simulink model "baseline_alt_vel_control"  (R2013a)
settings: Solver=FixedStepDiscrete  StartTime=0.0  StopTime=5  FixedStep=SampleTime  RelTol=1e-3
values from neighbouring files (symbols this model uses):
  ki_AT = 0.0017    [heading_gains.m]
  ki_VT = 0.02    [heading_gains.m]
  kp_AT = 0.021    [heading_gains.m]
  kp_VT = 0.091    [heading_gains.m]
  LP_filter = [0 0.0392;1 -.9608]    [heading_gains.m]
undefined symbols (not defined in the file or in its folder): AC, DiscIntNeverNeededParam, OperatingPoint, SampleTime, theta_sat, TrimCondition
libraries: Actuator_Lib x2, simulink x1, Controller_Lib x1
settings Model: Creator=austinmurch  LastModifiedBy=descobar
settings DataIOCC: SignalLoggingSaveFormat=ModelDataLogs
settings OptimizationCC: InlineParams=on  ExpressionDepthLimit=2147483647  SimCompilerOptimization=On
settings DebuggingCC: FcnCallInpInsideContextMsg=UseLocalSettings  StrictBusMsg=Warning
settings HardwareCC: ProdLargestAtomicInteger=Long  ProdLargestAtomicFloat=Double  ProdIntDivRoundTo=Zero  ProdEndianess=BigEndian  ProdHWDeviceType=Freescale->32-bit PowerPC
settings GRTTargetCC: CombineOutputUpdateFcns=off  GRTInterface=on

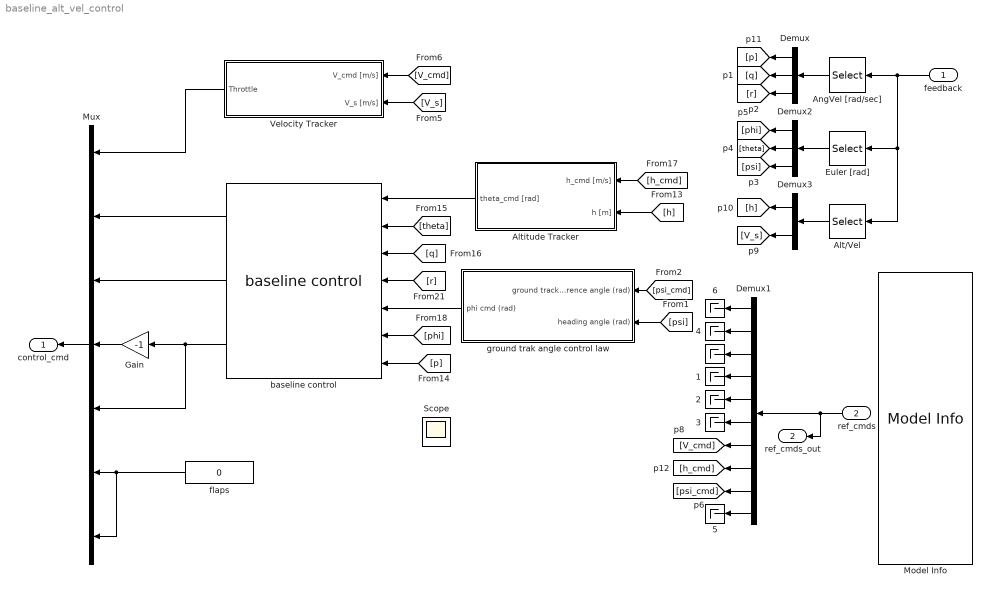
== system baseline_alt_vel_control ==
  feedback : Inport
  ref_cmds : Inport  Port=2
   {,1..6} (7 alike) : Terminator
  Alt/Vel : Selector  InputPortWidth=19  IndexOptions=Index vector (dialog)  Indices=[10:11]  OutputSizes=1
  Altitude Tracker : Subsystem
  AngVel [rad/sec] : Selector  InputPortWidth=19  IndexOptions=Index vector (dialog)  Indices=[4:6]  OutputSizes=1
  Demux : Demux  Outputs=3
  Demux1 : Demux  Outputs=[1 1 1 1 1 1 1 1 1 3]
  Demux2 : Demux  Outputs=3
  Demux3 : Demux  Outputs=2
  Euler [rad] : Selector  InputPortWidth=19  IndexOptions=Index vector (dialog)  Indices=[1:3]  OutputSizes=1
  Gain : Gain  Gain=-1
  Model Info : simulink/Model-Wide Utilities/Model Info  InitialBlockCM=None  BlockCM=None  Frame=on  DisplayStringWithTags=|  HorizontalTextAlignment=Center  LeftAlignmentValue=0.5  SourceBlockDiagram=baseline_alt_vel_control  TagMaxNumber=20
      | Ref Cmd Port Info
      | 
      | 1. phi_cmd
      | 2. theta_cmd
      | 3. psi_cmd
      | 4. p_cmd
      | 5. q_cmd
      | 6. r_cmd
      | 7. V_s_cmd
      | 8. h_cmd
      | 9. gndtrk_cmd
      | 10. aoa_cmd
      | 11. aos_cmd
      | 12. gamma_cmd
      | 13. signal_0
      | 14. signal_1
      | 15. signal_2
      | 16. signal_3
      | 17. signal_4
      | 18. signal_5
      | 19. signal_6
      | 20. signal_7
      | 21. signal_8
      | 22. signal_9
  Mux : Mux  Inputs=7
  Scope : Scope
  Velocity Tracker : Subsystem
  baseline control : Controller_Lib/baseline control  pitch=pitch_gains  roll=roll_gains  yaw_num=yaw_damper_num  yaw_den=yaw_damper_den
  flaps : Constant  Value=0
  ground trak angle control law : Subsystem
  control_cmd : Outport
  ref_cmds_out : Outport  Port=2
  wires:
  AngVel [rad/sec]/1 -> Demux/1
  Euler [rad]/1 -> Demux2/1
  Demux/1 -> [p]
  Demux/2 -> [q]
  Demux/3 -> [r]
  Demux2/3 -> [psi]
  feedback/1 -> AngVel [rad/sec]/1, Euler [rad]/1, Alt/Vel/1
  Demux2/2 -> [theta]
  Demux2/1 -> [phi]
  Alt/Vel/1 -> Demux3/1
  Mux/1 -> control_cmd/1
  Gain/1 -> Mux/4
  flaps/1 -> Mux/6, Mux/7
  Demux3/1 -> [h]
  Demux3/2 -> [V_s]
  Demux1/2 -> " 4"/1
  Demux1/7 -> [V_cmd]
  Demux1/5 -> " 2"/1
  Demux1/4 -> " 1"/1
  Demux1/3 -> " "/1
  Demux1/6 -> " 3"/1
  Demux1/8 -> [h_cmd]
  ref_cmds/1 -> ref_cmds_out/1, Demux1/1
  Demux1/9 -> [psi_cmd]
  [r] -> baseline control/4
  [q] -> baseline control/3
  [theta] -> baseline control/2
  [phi] -> baseline control/6
  [p] -> baseline control/7
  [h_cmd] -> Altitude Tracker/1(h_cmd [m/s])
  [h] -> Altitude Tracker/2(h [m])
  baseline control/1 -> Mux/2
  [V_cmd] -> Velocity Tracker/1(V_cmd [m/s])
  [V_s] -> Velocity Tracker/2(V_s [m/s])
  baseline control/3 -> Gain/1, Mux/5
  baseline control/2 -> Mux/3
  Altitude Tracker/1(theta_cmd [rad]) -> baseline control/1
  Velocity Tracker/1("Throttle ") -> Mux/1
  ground trak angle control law/1(phi cmd (rad)) -> baseline control/5
  Demux1/1 -> " 6"/1
  [psi] -> ground trak angle control law/2(heading angle (rad))
  Demux1/10 -> " 5"/1
  [psi_cmd] -> ground trak angle control law/1(ground track reference angle (rad))

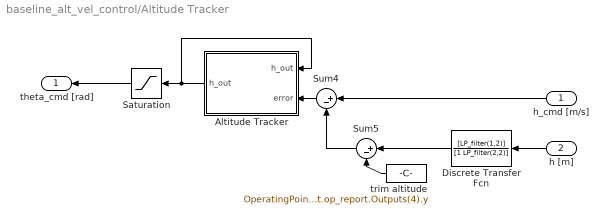
== system baseline_alt_vel_control/Altitude Tracker ==
  h_cmd [m/s] : Inport
  h [m] : Inport  Port=2
  Altitude Tracker : Subsystem
  Discrete Transfer Fcn : DiscreteTransferFcn  Numerator=[LP_filter(1,2)]  Denominator=[1 LP_filter(2,2)]  InitialStates=OperatingPoint.op_report.Outputs(4).y/LP_filter(1,2)  SampleTime=SampleTime
  Saturation : Saturate  UpperLimit=theta_sat*pi/180  LowerLimit=-theta_sat*pi/180  SampleTime=SampleTime
  Sum4 : Sum  Inputs=|+-  SampleTime=SampleTime
  Sum5 : Sum  Inputs=|+-  SampleTime=SampleTime
  trim altitude : Constant  Value=OperatingPoint.op_report.Outputs(4).y
  theta_cmd [rad] : Outport
  wires:
  h_cmd [m/s]/1 -> Sum4/1
  trim altitude/1 -> Sum5/2
  Sum5/1 -> Sum4/2
  h [m]/1 -> Discrete Transfer Fcn/1
  Discrete Transfer Fcn/1 -> Sum5/1
  Sum4/1 -> Altitude Tracker/2(error)
  Altitude Tracker/1(h_out) -> Saturation/1, Altitude Tracker/1(" h_out")
  Saturation/1 -> theta_cmd [rad]/1

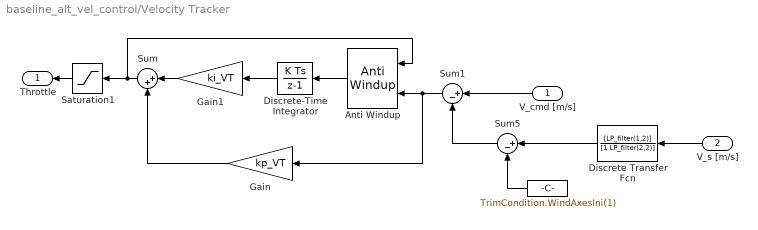
== system baseline_alt_vel_control/Velocity Tracker ==
  V_cmd [m/s] : Inport
  V_s [m/s] : Inport  Port=2
  "    " : Constant  Value=TrimCondition.WindAxesIni(1)
  Anti Windup : Actuator_Lib/Anti Windup  MAX_DEF=AC.Actuator.throttle.PosLim-TrimCondition.Inputs.throttle  MIN_DEF=AC.Actuator.throttle.NegLim-TrimCondition.Inputs.throttle  gain_sign=on
  Discrete Transfer Fcn : DiscreteTransferFcn  Numerator=[LP_filter(1,2)]  Denominator=[1 LP_filter(2,2)]  InitialStates=TrimCondition.target.V_s/LP_filter(1,2)  SampleTime=SampleTime
  Discrete-Time Integrator : DiscreteIntegrator  SampleTime=.02  ICPrevOutput=DiscIntNeverNeededParam  ICPrevScaledInput=DiscIntNeverNeededParam
  Gain : Gain  Gain=kp_VT
  Gain1 : Gain  Gain=ki_VT
  Saturation1 : Saturate  UpperLimit=AC.Actuator.throttle.PosLim-TrimCondition.Inputs.throttle  LowerLimit=AC.Actuator.throttle.NegLim-TrimCondition.Inputs.throttle  SampleTime=SampleTime
  Sum : Sum  Inputs=|++
  Sum1 : Sum  Inputs=|+-
  Sum5 : Sum  Inputs=|+-  SampleTime=SampleTime
  "Throttle " : Outport
  wires:
  Discrete-Time Integrator/1 -> Gain1/1
  Gain1/1 -> Sum/1
  Gain/1 -> Sum/2
  V_cmd [m/s]/1 -> Sum1/1
  Sum/1 -> Saturation1/1, Anti Windup/1
  "    "/1 -> Sum5/2
  Sum5/1 -> Sum1/2
  V_s [m/s]/1 -> Discrete Transfer Fcn/1
  Saturation1/1 -> "Throttle "/1
  Sum1/1 -> Anti Windup/2, Gain/1
  Anti Windup/1 -> Discrete-Time Integrator/1
  Discrete Transfer Fcn/1 -> Sum5/1

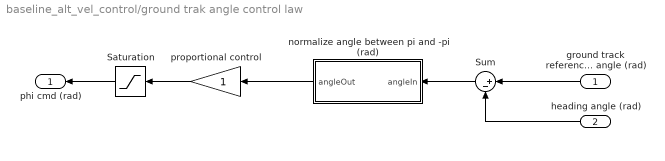
== system baseline_alt_vel_control/ground trak angle control law ==
  ground track reference angle (rad) : Inport
  heading angle (rad) : Inport  Port=2
  Saturation : Saturate  UpperLimit=40*pi/180  LowerLimit=-40*pi/180
  Sum : Sum  Inputs=|+-
  normalize angle between pi and -pi (rad) : MATLAB Function  TreatAsAtomicUnit=on
  proportional control : Gain
  phi cmd (rad) : Outport
  wires:
  ground track reference angle (rad)/1 -> Sum/1
  normalize angle between pi and -pi (rad)/1(angleOut) -> proportional control/1
  heading angle (rad)/1 -> Sum/2
  Sum/1 -> normalize angle between pi and -pi (rad)/1(angleIn)
  Saturation/1 -> phi cmd (rad)/1
  proportional control/1 -> Saturation/1

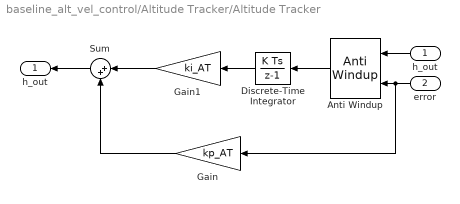
== system baseline_alt_vel_control/Altitude Tracker/Altitude Tracker ==
  " h_out" : Inport
  error : Inport  Port=2
  Anti Windup : Actuator_Lib/Anti Windup  MAX_DEF=AC.Actuator.elevator.PosLim-TrimCondition.Inputs.elevator  MIN_DEF=AC.Actuator.elevator.NegLim-TrimCondition.Inputs.elevator  gain_sign=on
  Discrete-Time Integrator : DiscreteIntegrator  SampleTime=.02  ICPrevOutput=DiscIntNeverNeededParam  ICPrevScaledInput=DiscIntNeverNeededParam
  Gain : Gain  Gain=kp_AT
  Gain1 : Gain  Gain=ki_AT
  Sum : Sum  Inputs=|++
  h_out : Outport
  wires:
  Discrete-Time Integrator/1 -> Gain1/1
  Gain1/1 -> Sum/1
  Sum/1 -> h_out/1
  Gain/1 -> Sum/2
  " h_out"/1 -> Anti Windup/1
  error/1 -> Anti Windup/2, Gain/1
  Anti Windup/1 -> Discrete-Time Integrator/1

== matlab function baseline_alt_vel_control/ground trak angle control law/normalize angle between pi and -pi (rad) ==
  data: angleOut output; angleIn input
function angleOut    = fcn(angleIn)
%#codegen
angleOut = angleIn;
if (angleOut < -pi)
   angleOut = 2*pi+angleOut ; 
end

if (angleOut > pi)
    angleOut = -2*pi+angleOut ; 
end
